simulink model "ex3aSim"  (R2023b)
settings: Solver=VariableStepAuto  StartTime=0.0  StopTime=100  RelTol=1e-3
values from neighbouring files (symbols this model uses):
  k = 5    [ex2.m]    (also in ex3a.m = 6)
settings Model: Creator=Bianca  LastModifiedBy=Bianca

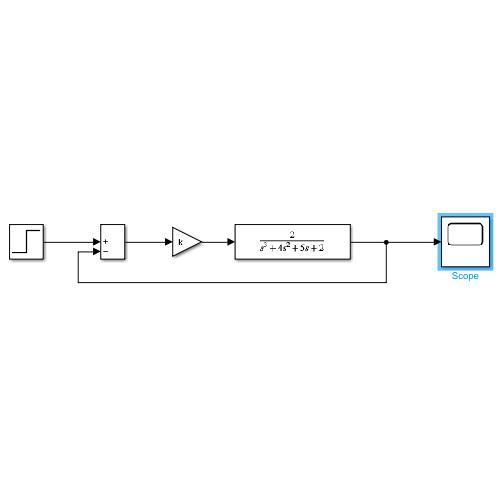
[thumbnail: Simulink's stored preview of the top-level diagram]
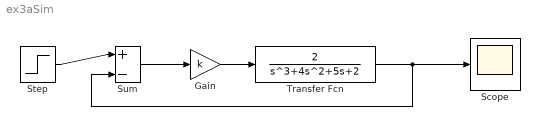
== system ex3aSim ==
  Gain : Gain  Gain=k
  Scope : Scope
  Step : Step  SampleTime=0
  Sum : Sum  Inputs=|+-
  Transfer Fcn : TransferFcn  Numerator=[0 0 0 2]  Denominator=[1 4 5 2]
  wires:
  Step/1 -> Sum/1
  Sum/1 -> Gain/1
  Gain/1 -> Transfer Fcn/1
  Transfer Fcn/1 -> Sum/2, Scope/1
